simulink library "dragTurbineVaryCpCt_ul"  (R2020a)
settings: Solver=VariableStepAuto  StartTime=0.0  StopTime=10.0  RelTol=1e-3
undefined symbols (not defined in the file): rho, tauLim, vcl
libraries: vrlib x2, simulink x1, localApparentWind_ul x1
settings Model: Creator=Ayaz  LastModifiedBy=adabney
settings DataIOCC: ReturnWorkspaceOutputs=off
settings DebuggingCC: ArithmeticOperatorsInVariantConditions=warning
settings SFSimCC: CustomCodeUndefinedFunction=UseInterfaceOnly

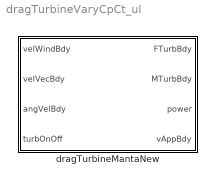
== system dragTurbineVaryCpCt_ul ==
  dragTurbineMantaNew : Subsystem  TreatAsAtomicUnit=on  mask{rho_fluid=rho, turb_struct=vcl.turb1}
      mask prompts: rho_fluid "Fluid density"; turb_struct "Turbines structure"

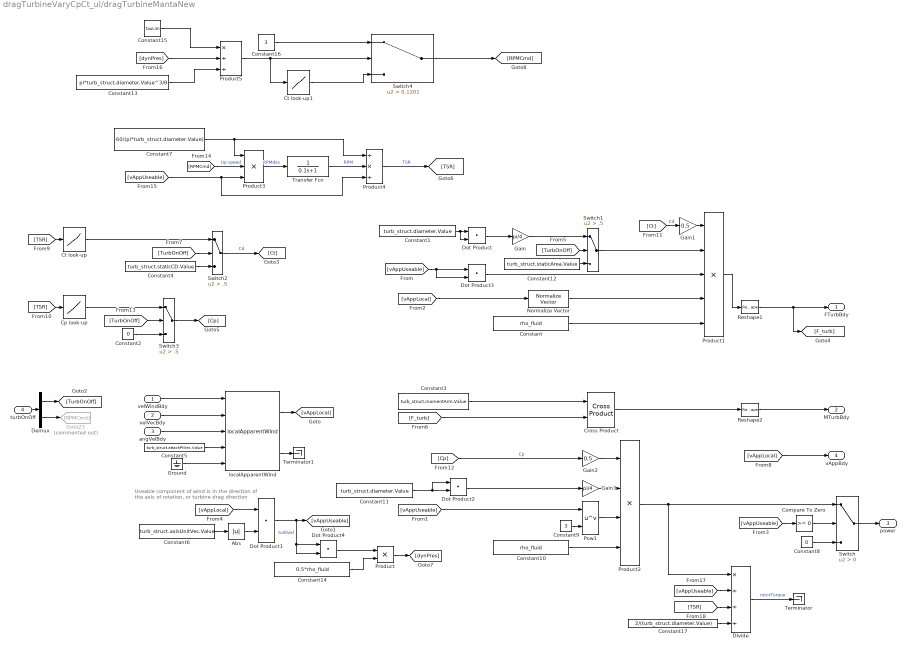
== system dragTurbineVaryCpCt_ul/dragTurbineMantaNew ==
  note: Useable component of wind is in the direction of
      | the axis of rotation, or turbine drag direction
  velWindBdy : Inport
  velVecBdy : Inport  Port=2
  angVelBdy : Inport  Port=3
  turbOnOff : Inport  Port=4
  Abs : Abs
  Compare To Zero : simulink/Logic and Bit Operations/Compare To Zero  relop=>=  OutDataTypeStr=boolean
  Constant : Constant  Value=rho_fluid
  Constant1 : Constant  Value=turb_struct.diameter.Value  VectorParams1D=off
  Constant10 : Constant  Value=rho_fluid
  Constant11 : Constant  Value=turb_struct.diameter.Value  VectorParams1D=off
  Constant12 : Constant  Value=turb_struct.staticArea.Value  VectorParams1D=off
  Constant13 : Constant  Value=pi*turb_struct.diameter.Value^3/8
  Constant14 : Constant  Value=0.5*rho_fluid
  Constant15 : Constant  Value=tauLim
  Constant16 : Constant  Value=3
  Constant17 : Constant  Value=2/(turb_struct.diameter.Value)
  Constant2 : Constant  Value=0
  Constant3 : Constant  Value=turb_struct.momentArm.Value
  Constant4 : Constant  Value=turb_struct.staticCD.Value
  Constant5 : Constant  Value=turb_struct.attachPtVec.Value
  Constant6 : Constant  Value=turb_struct.axisUnitVec.Value
  Constant7 : Constant  Value=60/(pi*turb_struct.diameter.Value)
  Constant8 : Constant  Value=0
  Constant9 : Constant  Value=3
  Cp look-up : Lookup_n-D  NumberOfTableDimensions=1  BreakpointsForDimension1=turb_struct.RPMref.Value  Table=turb_struct.CpLookup.Value  InternalRulePriority=Speed  RndMeth=Simplest  InputSameDT=on
  Cross Product : vrlib/Utilities/Cross Product
  Ct look-up : Lookup_n-D  NumberOfTableDimensions=1  BreakpointsForDimension1=turb_struct.RPMref.Value  Table=turb_struct.CtLookup.Value  InternalRulePriority=Speed  RndMeth=Simplest  InputSameDT=on
  Ct look-up1 : Lookup_n-D  NumberOfTableDimensions=1  BreakpointsForDimension1=turb_struct.torqueCoefLookup.Value(end:-1:1,2)  BreakpointsForDimension1Max=.1201  Table=turb_struct.torqueCoefLookup.Value(end:-1:1,1)  TableMin=3  InternalRulePriority=Speed  RndMeth=Simplest  InputSameDT=on
  Demux : Demux  Outputs=2
  Divide : Product  Inputs=*///
  Dot Product{,1..4} (5 alike) : DotProduct  InputSameDT=on  OutDataTypeStr=Inherit: Inherit via internal rule
  Gain : Gain  Gain=pi/4
  Gain1 : Gain  Gain=0.5
  Gain2 : Gain  Gain=0.5
  Gain3 : Gain  Gain=pi/4
  Goto23 : Goto  Commented=on  GotoTag=RPMCmd
  Ground : Ground
  Normalize Vector : vrlib/Utilities/Normalize Vector  maxzero=0
  Pow1 : Math  Operator=pow  SignedPower=on  RndMeth=Zero  SaturateOnIntegerOverflow=on
  Product : Product
  Product1 : Product  Inputs=5
  Product2 : Product  Inputs=4
  Product3 : Product  Inputs=3
  Product4 : Product  Inputs=/*/
  Product5 : Product  Inputs=*//
  Reshape1 : Reshape  OutputDimensionality=Column vector (2-D)
  Reshape2 : Reshape  OutputDimensionality=Column vector (2-D)
  Switch : Switch  Criteria=u2 > Threshold
  Switch1 : Switch  Criteria=u2 > Threshold  Threshold=.5
  Switch2 : Switch  Criteria=u2 > Threshold  Threshold=.5
  Switch3 : Switch  Criteria=u2 > Threshold  Threshold=.5
  Switch4 : Switch  Criteria=u2 > Threshold  Threshold=0.1201
  Terminator : Terminator
  Terminator1 : Terminator
  Transfer Fcn : TransferFcn  Denominator=[0.1 1]
  localApparentWind : localApparentWind_ul/localApparentWind  SystemSampleTime=-1  Latency=0  AutoFrameSizeCalculation=off
  FTurbBdy : Outport  PortDimensions=[3,1]  VectorParamsAs1DForOutWhenUnconnected=off
  MTurbBdy : Outport  Port=2  PortDimensions=[3,1]  VectorParamsAs1DForOutWhenUnconnected=off
  power : Outport  Port=3  PortDimensions=[1,1]  VectorParamsAs1DForOutWhenUnconnected=off
  vAppBdy : Outport  Port=4  PortDimensions=[3,1]  VectorParamsAs1DForOutWhenUnconnected=off
  wires:
  Gain3/1 -> Product2/2
  Constant11/1 -> Dot Product2/1, Dot Product2/2
  Dot Product2/1 -> Gain3/1
  [vAppUseable] -> Pow1/1
  [vAppLocal] -> Dot Product1/1
  Constant8/1 -> Switch/3
  [vAppUseable] -> Compare To Zero/1
  Compare To Zero/1 -> Switch/2
  Switch/1 -> power/1
  Pow1/1 -> Product2/3
  Gain2/1 -> Product2/1
  Constant10/1 -> Product2/4
  Constant/1 -> Product1/5
  Gain1/1 -> Product1/1
  Dot Product1/1 -> Dot Product4/2, Dot Product4/1, [vAppUseable]  "turbVel"
  Constant9/1 -> Pow1/2
  Normalize Vector/1 -> Product1/4
  [vAppUseable] -> Dot Product3/2, Dot Product3/1
  Constant6/1 -> Abs/1
  Constant5/1 -> localApparentWind/4
  localApparentWind/1 -> [vAppLocal]
  velWindBdy/1 -> localApparentWind/1
  angVelBdy/1 -> localApparentWind/3
  velVecBdy/1 -> localApparentWind/2
  Reshape2/1 -> MTurbBdy/1
  Reshape1/1 -> [F_turb], FTurbBdy/1
  [F_turb] -> Cross Product/2
  Constant3/1 -> Cross Product/1
  Product1/1 -> Reshape1/1
  Cross Product/1 -> Reshape2/1
  Ground/1 -> localApparentWind/5
  localApparentWind/2 -> Terminator1/1
  Abs/1 -> Dot Product1/2
  [vAppLocal] -> Normalize Vector/1
  [Cp] -> Gain2/1  "Cp"
  [vAppLocal] -> vAppBdy/1
  [TurbOnOff] -> Switch2/2
  turbOnOff/1 -> Demux/1
  Demux/1 -> [TurbOnOff]
  Demux/2 -> Goto23/1
  Switch1/1 -> Product1/2
  [TSR] -> Ct look-up/1
  [TSR] -> Cp look-up/1
  [TurbOnOff] -> Switch1/2
  Constant1/1 -> Dot Product/2, Dot Product/1
  Dot Product/1 -> Gain/1
  [TurbOnOff] -> Switch3/2
  Constant2/1 -> Switch3/3
  Switch3/1 -> [Cp]
  Cp look-up/1 -> Switch3/1
  [Ct] -> Gain1/1  "Cd"
  Constant4/1 -> Switch2/3
  Ct look-up/1 -> Switch2/1
  Switch2/1 -> [Ct]  "Cd"
  Constant12/1 -> Switch1/3
  Gain/1 -> Switch1/1
  Dot Product3/1 -> Product1/3
  [vAppUseable] -> Product4/3, Product3/3
  [RPMCmd] -> Product3/2  "tip speed"
  Constant7/1 -> Product3/1, Product4/1
  Product3/1 -> Transfer Fcn/1  "RPMdes"
  Transfer Fcn/1 -> Product4/2  "RPM"
  Product4/1 -> [TSR]  "TSR"
  Dot Product4/1 -> Product/1
  Constant14/1 -> Product/2
  Product/1 -> [dynPres]
  Constant15/1 -> Product5/1
  [dynPres] -> Product5/2
  Constant13/1 -> Product5/3
  Product5/1 -> Ct look-up1/1, Switch4/2
  Constant16/1 -> Switch4/1
  Ct look-up1/1 -> Switch4/3
  Switch4/1 -> [RPMCmd]
  Product2/1 -> Divide/1, Switch/1
  [vAppUseable] -> Divide/2
  [TSR] -> Divide/3
  Constant17/1 -> Divide/4
  Divide/1 -> Terminator/1  "rotorTorque"
